simulink model "levitador"  (R2019b)
settings: Solver=VariableStepAuto  StartTime=0.0  StopTime=10  RelTol=1e-3
undefined symbols (not defined in the file): eo, g, L, M, R, x10, x20, x30
settings Model: Creator=l53  LastModifiedBy=l53

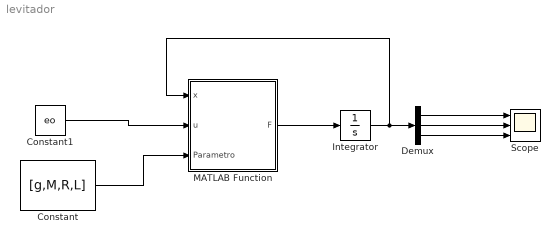
== system levitador ==
  Constant : Constant  Value=[g,M,R,L]
  Constant1 : Constant  Value=eo
  Demux : Demux  Outputs=3
  Integrator : Integrator  InitialCondition=[x10;x20;x30]
  MATLAB Function : MATLAB Function  TreatAsAtomicUnit=on
  Scope : Scope  NumInputPorts=3
  wires:
  MATLAB Function/1(F) -> Integrator/1
  Constant/1 -> MATLAB Function/3(Parametro)
  Constant1/1 -> MATLAB Function/2(u)
  Integrator/1 -> Demux/1, MATLAB Function/1(x)
  Demux/1 -> Scope/1
  Demux/2 -> Scope/2
  Demux/3 -> Scope/3

== matlab function levitador/MATLAB Function ==
  data: x input; u input; F output; Parametro input
function F = fcn(x,u,Parametro)
x1 = x(1);
x2 = x(2);
x3 = x(3);
e = u;
g = Parametro(1);
M = Parametro(2);
R = Parametro(3);
L = Parametro(4);
f1 = x2;
f2 = g - x3^2/(M*x1);
f3 = -R*x3/L+e/L;

F = [f1;f2;f3]
